simulink model "SimpleLRcircuit"  (R2014a)
settings: Solver=ode5  StartTime=0.0  StopTime=5  FixedStep=0.1  RelTol=1e-3
settings Model: Creator=carld  LastModifiedBy=carld

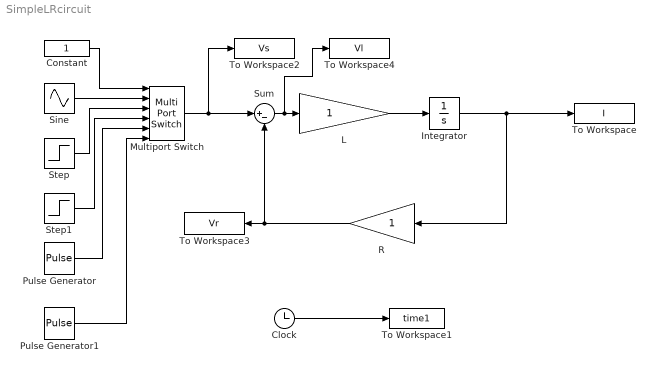
== system SimpleLRcircuit ==
  Clock : Clock
  Constant : Constant
  Integrator : Integrator
  L : Gain
  Multiport Switch : MultiPortSwitch  Inputs=5
  Pulse Generator : DiscretePulseGenerator  PulseType=Time based  Period=10  PhaseDelay=0.1
  Pulse Generator1 : DiscretePulseGenerator  PulseType=Time based  Amplitude=-1  Period=10  PhaseDelay=0.1
  R : Gain
  Sine : Sin  Frequency=2*pi*1  SampleTime=0
  Step : Step  Time=0.5  SampleTime=0
  Step1 : Step  Time=0.5  Before=1  After=0  SampleTime=0
  Sum : Sum  Inputs=|+-
  To Workspace : ToWorkspace  VariableName=I  SampleTime=-1
  To Workspace1 : ToWorkspace  VariableName=time1  SampleTime=-1
  To Workspace2 : ToWorkspace  VariableName=Vs  SampleTime=-1
  To Workspace3 : ToWorkspace  VariableName=Vr  SampleTime=-1
  To Workspace4 : ToWorkspace  VariableName=Vl  SampleTime=-1
  wires:
  R/1 -> Sum/2, To Workspace3/1
  Clock/1 -> To Workspace1/1
  Sum/1 -> To Workspace4/1, L/1
  L/1 -> Integrator/1
  Integrator/1 -> R/1, To Workspace/1
  Multiport Switch/1 -> To Workspace2/1, Sum/1
  Sine/1 -> Multiport Switch/2
  Constant/1 -> Multiport Switch/1
  Step/1 -> Multiport Switch/3
  Step1/1 -> Multiport Switch/4
  Pulse Generator/1 -> Multiport Switch/5
  Pulse Generator1/1 -> Multiport Switch/6
